simulink model "idhp_model_heart_realtime_syn"  (R2014a)
settings: Solver=FixedStepDiscrete  StartTime=0.0  StopTime=100  FixedStep=0.01  RelTol=1e-3
values from neighbouring files (symbols this model uses):
  Atr_refrD = 50    [const.m]
  AV_alpha = 150    [const.m]
  AV_anteDMin = 50    [const.m]
  AV_beta = 250    [const.m]
  AV_delta = 10    [const.m]
  AV_k4 = 0.03    [const.m]
  AV_refrDMin = 50    [const.m]
  AV_retroDMin = 100    [const.m]
  AV_tauC = 100    [const.m]
  AV_theta = 10    [const.m]
  AV_tr = 500    [const.m]
  AV_Vr = -90    [const.m]
  AV_Vt = -40    [const.m]
  PM_TAVI = 150    [const.m]
  PM_TLRI = 1000    [const.m]
  PM_TPVAB = 50    [const.m]
  PM_TPVARP = 250    [const.m]
  PM_TURI = 500    [const.m]
  PM_TVRP = 320    [const.m]
  RA_anteD = 30    [const.m]
  RA_retroD = 30    [const.m]
  RV_anteD = 50    [const.m]
  RV_retroD = 50    [const.m]
  SA_d = 850    [const.m]
  SA_dV = 50    [const.m]
  SA_ectopD = 10400    [const.m]
  SA_ectopdV = 50    [const.m]
  SA_noiseD = 1.0E+6    (= 1000000)    [const.m]
  VRG_d = 3000    [const.m]
  VRG_ectopD = 30450    [const.m]
  VRG_noiseD = 1.0E+6    (= 1000000)    [const.m]
  Vtr_refrD = 200    [const.m]
libraries: simulink x4
settings Model: Creator=alexandru  LastModifiedBy=barbot
settings DataIOCC: LimitDataPoints=off  SaveOutput=off  SignalLogging=off  DSMLogging=off  SaveTime=off
settings HardwareCC: TargetBitPerLong=64  TargetBitPerPointer=64  TargetLongLongMode=on  TargetIntDivRoundTo=Zero  TargetEndianess=LittleEndian  TargetWordSize=64  TargetHWDeviceType=MATLAB Host  ProdEqTarget=off
settings RTWCC: SystemTargetFile=rsim.tlc  GenCodeOnly=on  PackageGeneratedCodeAndArtifacts=on  PackageName=idhp_model_heart_realtime  TemplateMakefile=rsim_default_tmf  Description=Rapid Simulation Target  ProcessScript=rsim_make_rtw_hook
settings RSimTargetCC: ERTMultiwordTypeDef=System defined  ERTMultiwordLength=256  EnableShiftOperators=on

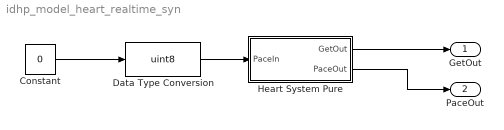
== system idhp_model_heart_realtime_syn ==
  Constant : Constant  Value=0
  Data Type Conversion : DataTypeConversion  OutDataTypeStr=uint8
  Heart System Pure : Subsystem
  GetOut : Outport
  PaceOut : Outport  Port=2
  wires:
  Data Type Conversion/1 -> Heart System Pure/1(PaceIn)
  Heart System Pure/1(GetOut) -> GetOut/1
  Heart System Pure/2(PaceOut) -> PaceOut/1
  Constant/1 -> Data Type Conversion/1

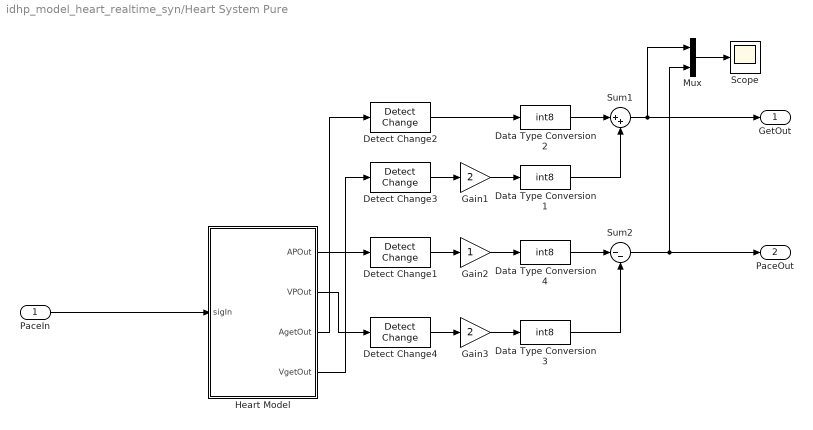
== system idhp_model_heart_realtime_syn/Heart System Pure ==
  PaceIn : Inport
  Data Type Conversion{1..4} (4 alike) : DataTypeConversion  OutDataTypeStr=int8
  Detect Change1 : simulink/Logic and Bit Operations/Detect Change  vinit=0  InputProcessing=Inherited  OutDataTypeStr=uint8
  Detect Change2 : simulink/Logic and Bit Operations/Detect Change  vinit=0  InputProcessing=Inherited  OutDataTypeStr=uint8
  Detect Change3 : simulink/Logic and Bit Operations/Detect Change  vinit=0  InputProcessing=Inherited  OutDataTypeStr=boolean
  Detect Change4 : simulink/Logic and Bit Operations/Detect Change  vinit=0  InputProcessing=Inherited  OutDataTypeStr=uint8
  Gain1 : Gain  Gain=2
  Gain2 : Gain
  Gain3 : Gain  Gain=2
  Heart Model : Stateflow chart  Priority=1  TreatAsAtomicUnit=on
  Mux : Mux  Inputs=2
  Scope : Scope
  Sum1 : Sum  Inputs=|++
  Sum2 : Sum  Inputs=|--
  GetOut : Outport
  PaceOut : Outport  Port=2
  wires:
  Detect Change3/1 -> Gain1/1
  Gain1/1 -> Data Type Conversion1/1
  Sum1/1 -> Mux/1, GetOut/1
  Data Type Conversion1/1 -> Sum1/2
  Detect Change2/1 -> Data Type Conversion2/1
  Data Type Conversion2/1 -> Sum1/1
  Heart Model/1(APOut) -> Detect Change1/1
  Heart Model/2(VPOut) -> Detect Change4/1
  Detect Change4/1 -> Gain3/1
  Gain3/1 -> Data Type Conversion3/1
  Data Type Conversion3/1 -> Sum2/2
  Data Type Conversion4/1 -> Sum2/1
  Sum2/1 -> PaceOut/1, Mux/2
  PaceIn/1 -> Heart Model/1(sigIn)
  Heart Model/4(VgetOut) -> Detect Change3/1
  Heart Model/3(AgetOut) -> Detect Change2/1
  Mux/1 -> Scope/1
  Detect Change1/1 -> Gain2/1
  Gain2/1 -> Data Type Conversion4/1

== stateflow chart idhp_model_heart_realtime_syn/Heart System Pure/Heart Model ==
  state Heart
    state A_dV [parallel]
      settings: executionOrder=13
      state a_dVLow
      state a_dvHigh
      (default) -> a_dVLow
      a_dVLow -> a_dvHigh [order 1] : a_dVSetHigh
      a_dVLow -> a_dVLow [order 2] : tr_AVJ
          | {send(AVJAnteReached,AVJ);}
      a_dvHigh -> a_dvHigh [order 2] : tr_AVJ
          | {send(AVJAnteReachedHigh,AVJ);}
      a_dvHigh -> a_dVLow [order 1] : a_dVSetLow
    state SANodeEctopic [parallel]
      settings: executionOrder=2
      state q0
      (default) -> Heart.SANodeEctopic.q0
      Heart.SANodeEctopic.q0 -> Heart.SANodeEctopic.q0 : after(SA_ectopD, msec)
          | {send(Abeat,Atrium);
          | send(a_dVSetHigh,A_dV);}
    state AtrNoiseGenerator [parallel]
      settings: executionOrder=1
      state q0
      (default) -> Heart.AtrNoiseGenerator.q0
      Heart.AtrNoiseGenerator.q0 -> Heart.AtrNoiseGenerator.q0 : after(SA_noiseD, msec)
          | {send(Aget,PVARP);}
    state RAConductor [parallel]
      settings: executionOrder=6
      state Empty
      state Ante
      state Retro
      (default) -> Heart.RAConductor.Empty
      Heart.RAConductor.Empty -> Heart.RAConductor.Ante [order 1] : arg
      Heart.RAConductor.Ante -> Heart.RAConductor.Empty [order 1] : retroAVJ
      Heart.RAConductor.Empty -> Heart.RAConductor.Retro [order 2] : retroAVJ
      Heart.RAConductor.Retro -> Heart.RAConductor.Empty [order 1] : arg
      Heart.RAConductor.Retro -> Heart.RAConductor.Empty [order 2] : after(RA_retroD,msec)
          | {send(AtrRetroReached,...
          | Atrium);}
      Heart.RAConductor.Ante -> Heart.RAConductor.Empty [order 2] : after(RA_anteD,msec)
          | {send(tr_AVJ,A_dV);}
    state AVJOut [parallel]
      settings: executionOrder=4
      state Empty
      state Ante
      state Retro
      (default) -> Heart.AVJOut.Empty
      Heart.AVJOut.Ante -> Heart.AVJOut.Empty : after(AVJDelay(avj_tRec,...
          | AV_anteDMin),msec)
          | {send(anteAVJ,RVConductor);}
      Heart.AVJOut.Empty -> Heart.AVJOut.Ante [order 1] : AVJAnteExit
      Heart.AVJOut.Retro -> Heart.AVJOut.Empty : after(AVJDelay(avj_tRec,...
          | AV_retroDMin),msec)
          | {send(retroAVJ,...
          | RAConductor);}
      Heart.AVJOut.Empty -> Heart.AVJOut.Retro [order 2] : AVJRetroExit
    state VRGEctopic [parallel]
      settings: executionOrder=10
      state q0
      (default) -> Heart.VRGEctopic.q0
      Heart.VRGEctopic.q0 -> Heart.VRGEctopic.q0 : after(VRG_ectopD, msec)
          | {send(Vbeat,Ventricle);}
    state RVConductor [parallel]
      settings: executionOrder=5
      state Empty
      state Ante
      state Retro
      (default) -> Heart.RVConductor.Empty
      Heart.RVConductor.Empty -> Heart.RVConductor.Ante [order 1] : anteAVJ
      Heart.RVConductor.Empty -> Heart.RVConductor.Retro [order 2] : vrg
      Heart.RVConductor.Ante -> Heart.RVConductor.Empty [order 1] : vrg
      Heart.RVConductor.Ante -> Heart.RVConductor.Empty [order 2] : after(RV_anteD,msec)
          | {send(VtrAnteReached,...
          | Ventricle);}
      Heart.RVConductor.Retro -> Heart.RVConductor.Empty [order 1] : anteAVJ
      Heart.RVConductor.Retro -> Heart.RVConductor.Empty [order 2] : after(RV_retroD,msec)
          | {send(AVJRetroReached,...
          | AVJ);}
    state VtrNoiseGenerator [parallel]
      settings: executionOrder=3
      state q0
      Heart.VtrNoiseGenerator.q0 -> Heart.VtrNoiseGenerator.q0 : after(VRG_noiseD, msec)
          | {send(Vget,VRP);}
      (default) -> Heart.VtrNoiseGenerator.q0
    state SANode [parallel]
      settings: executionOrder=7
      state Wait4ABeat
      state Wait4ASynch
      (default) -> Wait4ABeat
      Wait4ABeat -> Wait4ASynch [order 2] : after(SA_d, msec)
          | {send(Abeat,Atrium);
          | send(a_dVSetLow,A_dV);
          | }
      Wait4ABeat -> Wait4ABeat [order 1] : NextAtrBeat
      Wait4ASynch -> Wait4ABeat : NextAtrBeat
    state VRG [parallel]
      settings: executionOrder=11
      state Wait4VBeat
      state Wait4VSynch
      (default) -> Wait4VBeat
      Wait4VBeat -> Wait4VSynch [order 2] : after(VRG_d, msec)
          | {send(Vbeat,Ventricle);}
      Wait4VSynch -> Wait4VBeat : NextVtrBeat
      Wait4VBeat -> Wait4VBeat [order 1] : NextVtrBeat
    state AVJ [parallel]
      settings: executionOrder=12
      state Recovery
      state Ante
      state Refractory
      state Retro
      (default) -> Recovery : {avj_t4=timeToDep(AV_Vr);
          | ctime=0;
          | recoverylast=0;
          | refractorylast=0;
          | }
      Heart.AVJ.Ante -> Heart.AVJ.Refractory : after(avj_t4,msec)
          | {ctime=ctime+temporalCount(msec);
          | avj_tRec=(ctime-recoverylast);
          | send(AVJAnteExit,AVJOut);
          | avj_refr_0=initRefrPeriod(avj_tRec);
          | avj_refr=avj_refr_0;
          | refractorylast=ctime;}
      Recovery -> Heart.AVJ.Ante [order 1] : AVJAnteReached{
          | ctime=ctime+temporalCount(msec);
          | avj_t4 = timeToDep(AV_Vr+ ...
          | (ctime-recoverylast)*AV_k4 + SA_dV);
          | }
      Recovery -> Heart.AVJ.Ante [order 3] : AVJAnteReachedHigh{
          | ctime=ctime+temporalCount(msec);
          | avj_t4 = timeToDep(AV_Vr+...
          | (ctime-recoverylast)*AV_k4 + SA_ectopdV);
          | }
      Heart.AVJ.Refractory -> Recovery [order 4] : after(avj_refr,msec){
          | ctime=ctime+temporalCount(msec);
          | avj_t4=timeToDep(AV_Vr);
          | recoverylast=ctime;
          | }
      Recovery -> Heart.AVJ.Retro [order 4] : AVJRetroReached{
          | ctime=ctime+temporalCount(msec);
          | }
      Recovery -> Heart.AVJ.Refractory [order 2] : after(avj_t4,msec){
          | ctime=ctime+temporalCount(msec);
          | avj_tRec=avj_t4;
          | avj_refr_0=initRefrPeriod(avj_tRec);
          | avj_refr=avj_refr_0;
          | refractorylast=ctime;}
      Heart.AVJ.Refractory -> Heart.AVJ.Refractory [order 3] : AVJAnteReachedHigh
          | {ctime=ctime+temporalCount(msec);
          | avj_refr=avj_refr-(ctime - refractorylast)+...
          | modulateRefrAnte((ctime - refractorylast),...
          | avj_refr_0,SA_ectopdV);
          | refractorylast=ctime;
          | }
      Heart.AVJ.Refractory -> Heart.AVJ.Refractory [order 1] : AVJAnteReached
          | {ctime=ctime+temporalCount(msec);
          | avj_refr=avj_refr-(ctime - refractorylast)+...
          | modulateRefrAnte((ctime - refractorylast),...
          | avj_refr_0,SA_dV);
          | refractorylast=ctime;}
      Heart.AVJ.Refractory -> Heart.AVJ.Refractory [order 2] : AVJRetroReached
          | {ctime=ctime+temporalCount(msec);
          | avj_refr=avj_refr-(ctime - refractorylast)+...
          | modulateRefrRetro((ctime - refractorylast),...
          | avj_refr_0);
          | refractorylast=ctime;}
      Heart.AVJ.Retro -> Heart.AVJ.Refractory : {send(AVJRetroExit,AVJOut);
          | ctime=ctime+temporalCount(msec);
          | avj_tRec=ctime-recoverylast;
          | avj_refr_0=initRefrPeriod(avj_tRec);
          | avj_refr=avj_refr_0;
          | refractorylast=ctime;
          | }
    state Ventricle [parallel]
      settings: executionOrder=8
      state Excitable
      state Refractory
      state VsenseAnte
      state VSynch
      state Vsense
      state GenerateRetroWave
      (default) -> Heart.Ventricle.Refractory
      Heart.Ventricle.Refractory -> Heart.Ventricle.Excitable : after(Vtr_refrD,msec)
      Heart.Ventricle.Excitable -> Vsense [order 3] : Vbeat{VgetOut;}
      Heart.Ventricle.Excitable -> VsenseAnte [order 1] : VtrAnteReached{VgetOut;}
      VSynch -> Heart.Ventricle.Refractory : {send(NextVtrBeat,...
          | VRG);}
      Heart.Ventricle.Excitable -> GenerateRetroWave [order 2] : VP
          | {VPOut;}
      VsenseAnte -> VSynch : {send(Vget,VRP);}
      GenerateRetroWave -> VSynch : {send(vrg,RVConductor);}
      Vsense -> GenerateRetroWave : {send(Vget,VRP);}
    state Atrium [parallel]
      settings: executionOrder=9
      state Excitable
      state Refractory
      state ASynch
      state AsenseRetro
      state Asense
      state GenerateAnteWave
      (default) -> Heart.Atrium.Refractory
      Heart.Atrium.Excitable -> Asense [order 1] : Abeat{AgetOut;}
      Heart.Atrium.Refractory -> Heart.Atrium.Excitable : after(Atr_refrD,msec)
      Heart.Atrium.Excitable -> AsenseRetro [order 3] : AtrRetroReached{AgetOut;}
      ASynch -> Heart.Atrium.Refractory : {send(NextAtrBeat,...
          | SANode);}
      Heart.Atrium.Excitable -> GenerateAnteWave [order 2] : AP
          | {APOut;}
      AsenseRetro -> ASynch : {send(Aget,PVARP);}
      GenerateAnteWave -> ASynch : {send(arg,RAConductor);}
      Asense -> GenerateAnteWave : {send(Aget,PVARP);}
    state LRI [parallel]
      settings: executionOrder=14
      state LRI
      state ASensed
      Heart.LRI.LRI -> Heart.LRI.LRI [order 2] : after(PM_TLRI-PM_TAVI,msec){
          | send(AP,Atrium);
          | send(AP,AVI);
          | }
      Heart.LRI.LRI -> ASensed [order 3] : AS
      (default) -> Heart.LRI.LRI
      ASensed -> Heart.LRI.LRI : RLRI
      Heart.LRI.LRI -> Heart.LRI.LRI [order 1] : RLRI
    state URI [parallel]
      settings: executionOrder=15
      state URI
      state q1
      Heart.URI.URI -> Heart.URI.URI [order 1] : RURI
      (default) -> Heart.URI.URI
      Heart.URI.URI -> Heart.URI.q1 [order 2] : after(PM_TURI,msec){}
      Heart.URI.q1 -> Heart.URI.URI : {send(IncrClk,AVI);}
    state AVI [parallel]
      settings: executionOrder=16
      state Idle0
      state AVI0
      state WaitURI
      state Idle1
      state AVI1
      WaitURI -> Idle0 [order 1] : VS{send(RURI,URI);}
      AVI0 -> Idle0 [order 3] : VS{send(RURI,URI);}
      Idle0 -> AVI0 [order 2] : AP{send(RTAVI,TAVIcmp);}
      (default) -> Idle0
      AVI0 -> WaitURI [order 2] : TAVI
      Idle0 -> AVI0 [order 3] : AS{send(RTAVI,TAVIcmp);}
      AVI1 -> Idle0 [order 2] : TAVI{
          | send(RLRI,LRI);
          | send(VP,VRP);
          | send(VP,PVARP);
          | send(VP,Ventricle);
          | send(RURI,URI);
          | }
      AVI1 -> Idle0 [order 1] : VS{send(RURI,URI);}
      WaitURI -> Idle0 [order 2] : IncrClk{
          | send(RLRI,LRI);
          | send(VP,VRP);
          | send(VP,PVARP);
          | send(VP,Ventricle);
          | }
      AVI0 -> AVI1 [order 1] : IncrClk
      Idle0 -> Idle1 [order 1] : IncrClk
      Idle1 -> AVI1 [order 2] : AP{send(RTAVI,TAVIcmp);}
      Idle1 -> AVI1 [order 1] : AS{send(RTAVI,TAVIcmp);}
    state VRP [parallel]
      settings: executionOrder=17
      state Idle
      state VRP
      state Vsig
      Heart.VRP.VRP -> Heart.VRP.Idle : after(PM_TVRP,msec)
      (default) -> Heart.VRP.Idle
      Heart.VRP.Idle -> Heart.VRP.VRP [order 2] : VP
      Vsig -> Heart.VRP.Idle : {send(RLRI, LRI);
          | send(VS, AVI);
          | send(VS, PVARP);}
      Heart.VRP.Idle -> Vsig [order 1] : Vget
    state TAVIcmp [parallel]
      settings: executionOrder=18
      state q0
      state q1
      Heart.TAVIcmp.q0 -> Heart.TAVIcmp.q1 : after(PM_TAVI,msec){send(TAVI,AVI);}
      Heart.TAVIcmp.q1 -> Heart.TAVIcmp.q0 : RTAVI
      (default) -> Heart.TAVIcmp.q1
    state PVARP [parallel]
      settings: executionOrder=19
      state Idle
      state PVAB
      state Asig
      state PVARP
      Heart.PVARP.Idle -> PVAB [order 3] : VP
      Heart.PVARP.Idle -> PVAB [order 2] : VS
      (default) -> Heart.PVARP.Idle
      Heart.PVARP.PVARP -> Heart.PVARP.Idle : after(PM_TPVARP-...
          | PM_TPVAB,msec)
      Asig -> Heart.PVARP.Idle : {send(AS,LRI);
          | send(AS,AVI);
          | send(AS,TAVIcmp);}
      Heart.PVARP.Idle -> Asig [order 1] : Aget
      PVAB -> Heart.PVARP.PVARP : after(PM_TPVAB,msec)
  (default) -> Heart
  data: t function_output double; tRec function_input double; minDly function_input double; t function_output double; Vm function_input double; t function_output double; tRec function_input double; t function_input double; dT function_output double; t0 function_input double; t function_input double; t0 function_input double; dT function_output double; dV function_input double; Atr_refrD parameter; AV_alpha parameter; AV_anteDMin parameter; AV_beta parameter; AV_delta parameter; AV_k4 parameter; AV_refrDMin parameter; AV_retroDMin parameter; AV_tauC parameter; AV_theta parameter; AV_tr parameter; AV_Vr parameter; AV_Vt parameter; RA_anteD parameter; RA_retroD parameter; RV_anteD parameter; RV_retroD parameter; SA_d parameter; SA_dV parameter; SA_ectopD parameter; SA_ectopdV parameter; SA_noiseD parameter; VRG_d parameter; VRG_ectopD parameter; VRG_noiseD parameter; Vtr_refrD parameter; avj_tRec local double; sigIn input uint8; clk local double; PM_TAVI parameter; PM_TLRI parameter; PM_TPVAB parameter; PM_TPVARP parameter; PM_TURI parameter; PM_TVRP parameter; recoverylast local double; avj_t4 local double; ctime local double; avj_refr local double; avj_refr_0 local double; refractorylast local double
  events: Abeat local FUNCTION_CALL_EVENT; AtrRetroReached local FUNCTION_CALL_EVENT; arg local FUNCTION_CALL_EVENT; retroAVJ local FUNCTION_CALL_EVENT; AVJAnteReached local FUNCTION_CALL_EVENT; NextAtrBeat local FUNCTION_CALL_EVENT; AVJRetroReached local FUNCTION_CALL_EVENT; anteAVJ local FUNCTION_CALL_EVENT; vrg local FUNCTION_CALL_EVENT; VtrAnteReached local FUNCTION_CALL_EVENT; AVJRetroExit local FUNCTION_CALL_EVENT; AVJAnteExit local FUNCTION_CALL_EVENT; NextVtrBeat local FUNCTION_CALL_EVENT; Vbeat local FUNCTION_CALL_EVENT; AP local EITHER_EDGE_EVENT; VP local EITHER_EDGE_EVENT; APOut output EITHER_EDGE_EVENT; VPOut output EITHER_EDGE_EVENT; AS local RISING_EDGE_EVENT; VS local RISING_EDGE_EVENT; Aget local EITHER_EDGE_EVENT; Vget local EITHER_EDGE_EVENT; Aintrinsic local EITHER_EDGE_EVENT; Anoise local EITHER_EDGE_EVENT; Aretro local EITHER_EDGE_EVENT; Vintrinsic local EITHER_EDGE_EVENT; Vnoise local EITHER_EDGE_EVENT; Vante local EITHER_EDGE_EVENT; AgetOut output EITHER_EDGE_EVENT; VgetOut output EITHER_EDGE_EVENT; APElectr local RISING_EDGE_EVENT; VPElectr local EITHER_EDGE_EVENT; IncrClk local FUNCTION_CALL_EVENT; State local FUNCTION_CALL_EVENT; Clk0 local FUNCTION_CALL_EVENT; Clk1 local FUNCTION_CALL_EVENT; a_dVSetHigh local FUNCTION_CALL_EVENT; a_dVSetLow local FUNCTION_CALL_EVENT; tr_AVJ local FUNCTION_CALL_EVENT; AVJAnteReachedHigh local FUNCTION_CALL_EVENT; RLRI local FUNCTION_CALL_EVENT; TAVI local FUNCTION_CALL_EVENT; RTAVI local FUNCTION_CALL_EVENT; RURI local FUNCTION_CALL_EVENT
  function t  = AVJDelay(tRec,minDly):
    | function t  = AVJDelay(tRec,minDly)
    |     t = minDly+AV_alpha*exp(-tRec/AV_tauC);
    | end
  function t  = timeToDep(Vm):
    | function t  = timeToDep(Vm)
    |     t = max(0,(AV_Vt-Vm)/AV_k4);
    | end
  function t  = initRefrPeriod(tRec):
    | function t  = initRefrPeriod(tRec)
    |     t = AV_refrDMin + AV_beta*(1 - exp(-tRec/AV_tr));
    | end
  function dT  = modulateRefrRetro(t,t0):
    | 
    | function dT  = modulateRefrRetro(t,t0)
    |     dT = AV_refrDMin*power(t/t0,AV_theta);
    | end
  function dT  = modulateRefrAnte(t,t0,dV):
    | function dT  = modulateRefrAnte(t,t0,dV)
    |     %val1 = t/t0;
    |     %val2 = power(t/t0,avj_theta);
    |     dT = AV_refrDMin*power(t/t0,AV_theta)*power(min(1,dV/(AV_Vt-AV_Vr)),AV_delta);
    |     %fprintf(1,'%f %f\n', val1, val2);
    | end
